simulink model "WiperSysCtrlLab"  (R2022b)
settings: Solver=FixedStepDiscrete  StartTime=0.0  StopTime=10  FixedStep=0.1  MaxStep=0.1  RelTol=1e-3
libraries: simulink x1
settings Model: Creator=ahmed  LastModifiedBy=ahmed

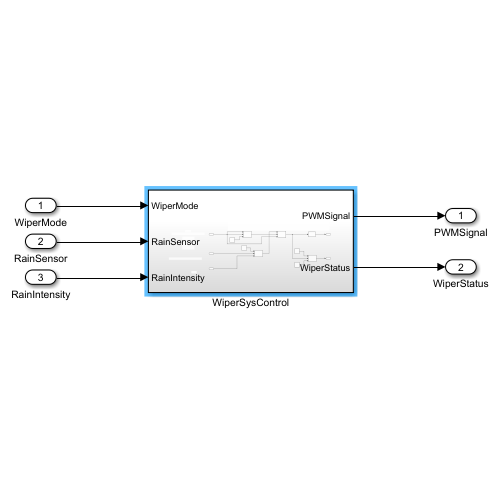
[thumbnail: Simulink's stored preview of the top-level diagram]
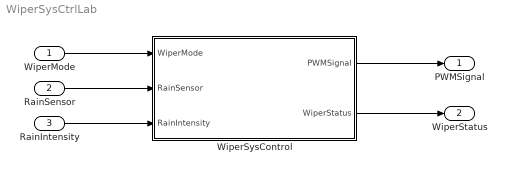
== system WiperSysCtrlLab ==
  WiperMode : Inport
  RainSensor : Inport  Port=2
  RainIntensity : Inport  Port=3
  WiperSysControl : Subsystem
  PWMSignal : Outport
  WiperStatus : Outport  Port=2
  wires:
  WiperSysControl/1(PWMSignal) -> PWMSignal/1
  WiperSysControl/2(WiperStatus) -> WiperStatus/1
  WiperMode/1 -> WiperSysControl/1(WiperMode)
  RainIntensity/1 -> WiperSysControl/3(RainIntensity)
  RainSensor/1 -> WiperSysControl/2(RainSensor)

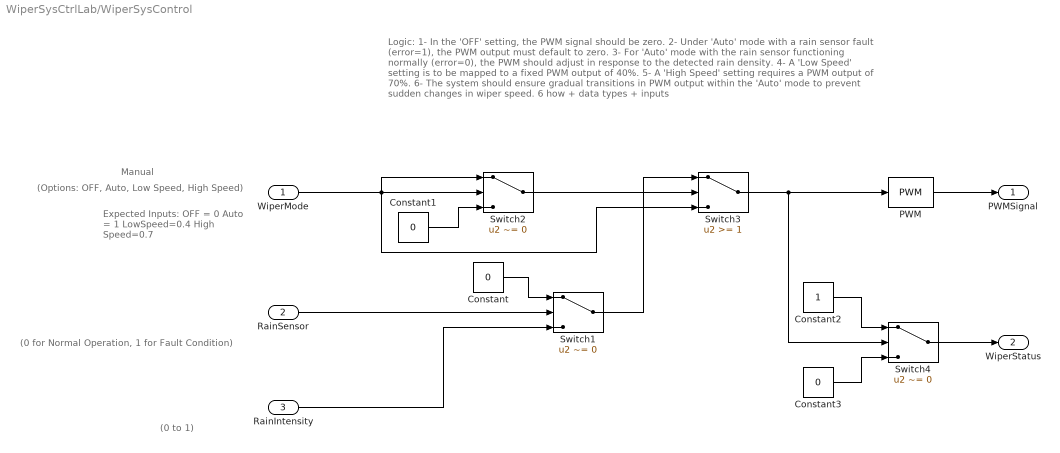
== system WiperSysCtrlLab/WiperSysControl ==
  note: Expected Inputs:
      | OFF = 0
      | Auto = 1
      | LowSpeed=0.4
      | High Speed=0.7
  note: (0 to 1)
  note: Manual
  note: Logic:
      | 1- In the 'OFF' setting, the PWM signal should be zero.
      | 2- Under 'Auto' mode with a rain sensor fault (error=1), the PWM output must default to zero.
      | 3- For 'Auto' mode with the rain sensor functioning normally (error=0), the PWM should adjust in response to the detected rain density.
      | 4- A 'Low Speed' setting is to be mapped to a fixed PWM output of 40%.
      | 5- A 'High Speed' setting requires a PWM output of 70%.
      | 6- The system should ensure gradual transitions in PWM output within the 'Auto' mode to prevent sudden changes in wiper speed.
      | 6 how + data types + inputs
  note: (0 for Normal Operation, 1 for Fault Condition)
  note: (Options: OFF, Auto, Low Speed, High Speed)
  WiperMode : Inport
  RainSensor : Inport  Port=2
  RainIntensity : Inport  Port=3
  Constant : Constant  Value=0
  Constant1 : Constant  Value=0
  Constant2 : Constant
  Constant3 : Constant  Value=0
  PWM : simulink/Discontinuities/PWM  DisableCoverage=on  Period=1  InitialDelay=0  DisallowZeroDutyCycle=off  RunAtFixedTimeIntervals=on  SampleTime=0.1
  Switch1 : Switch  Criteria=u2 ~= 0  SaturateOnIntegerOverflow=off  InputSameDT=off
  Switch2 : Switch  Criteria=u2 ~= 0  SaturateOnIntegerOverflow=off  InputSameDT=off
  Switch3 : Switch  Threshold=1  SaturateOnIntegerOverflow=off  InputSameDT=off
  Switch4 : Switch  Criteria=u2 ~= 0  SaturateOnIntegerOverflow=off  InputSameDT=off
  PWMSignal : Outport
  WiperStatus : Outport  Port=2
  wires:
  PWM/1 -> PWMSignal/1
  Switch2/1 -> Switch3/2
  Switch1/1 -> Switch3/1
  Constant3/1 -> Switch4/3
  WiperMode/1 -> Switch3/3, Switch2/1, Switch2/2
  Switch3/1 -> Switch4/2, PWM/1
  Constant2/1 -> Switch4/1
  Constant/1 -> Switch1/1
  Constant1/1 -> Switch2/3
  RainSensor/1 -> Switch1/2
  Switch4/1 -> WiperStatus/1
  RainIntensity/1 -> Switch1/3
